simulink model "Test_Ralenti_BO_End_New"  (R2024b)
settings: Solver=ode45  StartTime=0.0  StopTime=80  FixedStep=10e-3  MaxStep=0.01  RelTol=1e-5  AbsTol=1e-6
undefined symbols (not defined in the file): AaNeTest, AirMotTest, AirPapTest, AirPressureTest, AirTimeTest, Copti, EngineSpeedTest, EngineSpeedTimeTest, NeTest, NeTimeTest, PcolNeTest, SectionBpNeTest, table_rdt_AA, TorqueLosesTest, TorqueLosesTimeTest, vect_delta_AA
settings Model: Creator=a030141  LastModifiedBy=ramse
settings SolverCC: AutoScaleAbsTol=off  AlgebraicLoopSolver=TrustRegion
settings DataIOCC: SaveFormat=Array  SignalLoggingSaveFormat=ModelDataLogs  ReturnWorkspaceOutputs=off  SignalLoggingName=sigsOut
settings OptimizationCC: BlockReduction=off  BooleanDataType=off  InitFltsAndDblsToZero=on  LifeSpan=inf
settings DebuggingCC: SaveWithParameterizedLinksMsg=none  UnderspecifiedInitializationDetection=Classic  MergeDetectMultiDrivingBlocksExec=none  SignalResolutionControl=TryResolveAllWithWarning  MultiTaskDSMMsg=warning  MultiTaskCondExecSysMsg=none  FcnCallInpInsideContextMsg=warning  UnconnectedInputMsg=warning  UnconnectedOutputMsg=warning  UnconnectedLineMsg=warning  SFUnexpectedBacktrackingDiag=warning  SFNoUnconditionalDefaultTransitionDiag=warning  SFExecutionAtInitializationDiag=none  ArithmeticOperatorsInVariantConditions=warning
settings HardwareCC: ProdBitPerPointer=32  ProdBitPerSizeT=32  ProdBitPerPtrDiffT=32  ProdLargestAtomicFloat=None  ProdIntDivRoundTo=Undefined  ProdEndianess=Unspecified  ProdWordSize=32  ProdHWDeviceType=32-bit Generic  TargetUnknown=on
settings ModelReferenceCC: PropagateSignalLabelsOutOfModel=off
settings RTWCC: TemplateMakefile=grt_vc.tmf  GPUComputeCapability=3.5
settings CodeAppCC: StateflowObjectComments=on
settings GRTTargetCC: TargetFcnLib=ansi_tfl_tmw.mat  TargetLangStandard=C89/C90 (ANSI)  CombineOutputUpdateFcns=off  GRTInterface=on
settings ConfigComp: CovMetricSettings=dw  CovSaveCumulativeToWorkspaceVar=on  CovSaveSingleToWorkspaceVar=on

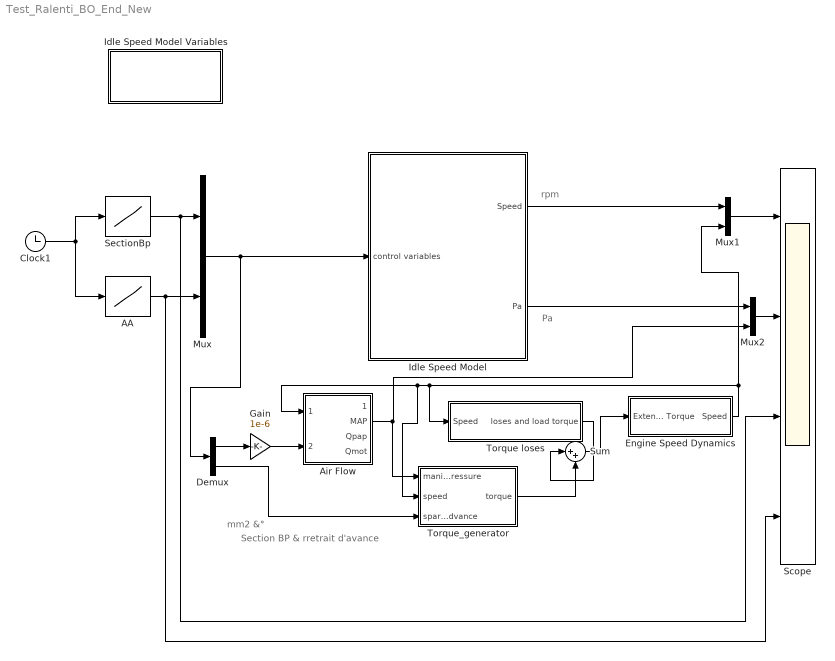
== system Test_Ralenti_BO_End_New ==
  note: Section BP & rretrait d'avance
  note: Pa
  note: rpm
  note: mm2 &°
  " Torque loses" : Subsystem
  AA : Lookup  InputValues=NeTimeTest  Table=AaNeTest
  Air Flow : Subsystem
  Clock1 : Clock
  Demux : Demux  Outputs=2
  Engine Speed Dynamics : Subsystem
  Gain : Gain  Gain=1e-6
  Idle Speed Model : Subsystem
      mask Display: disp('ENGINE MODEL\nLF -> event stroke')
  Idle Speed Model Variables : Subsystem
      mask Display: disp('Load\nDisturbances')
  Mux : Mux  Inputs=2
  Mux1 : Mux  Inputs=2
  Mux2 : Mux  Inputs=2
  Scope : Scope  NumInputPorts=4
  SectionBp : Lookup  InputValues=NeTimeTest  Table=SectionBpNeTest
  Sum : Sum  Inputs=|++
  Torque_generator : Subsystem
  wires:
  Mux/1 -> Demux/1, Idle Speed Model/1(control variables)
  SectionBp/1 -> Mux/1, Scope/3
  AA/1 -> Mux/2, Scope/4
  Clock1/1 -> SectionBp/1, AA/1
  Idle Speed Model/1(Speed) -> Mux1/1
  Mux1/1 -> Scope/1
  Idle Speed Model/2(Pa) -> Mux2/1
  Mux2/1 -> Scope/2
  Air Flow/2(MAP) -> Torque_generator/1(manifold pressure), Mux2/2
  Demux/1 -> Gain/1
  Gain/1 -> Air Flow/2(Bypass)
  Demux/2 -> Torque_generator/3(spark advance)
  Torque_generator/1(torque) -> Sum/2
  " Torque loses"/1(loses and load torque) -> Sum/1
  Sum/1 -> Engine Speed Dynamics/1(Extended Torque)
  Engine Speed Dynamics/1(Speed) -> " Torque loses"/1(Speed), Torque_generator/2(speed), Air Flow/1(Speed), Mux1/2

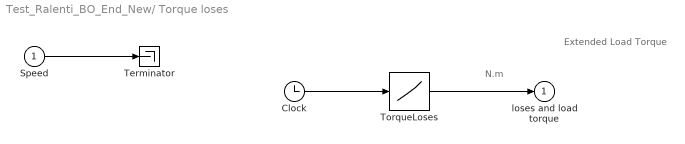
== system Test_Ralenti_BO_End_New/ Torque loses ==
  note: N.m
  note: Extended Load Torque
  Speed : Inport
  Clock : Clock
  Terminator : Terminator
  TorqueLoses : Lookup  InputValues=TorqueLosesTimeTest  Table=TorqueLosesTest
  loses and load torque : Outport
  wires:
  Clock/1 -> TorqueLoses/1
  TorqueLoses/1 -> loses and load torque/1
  Speed/1 -> Terminator/1

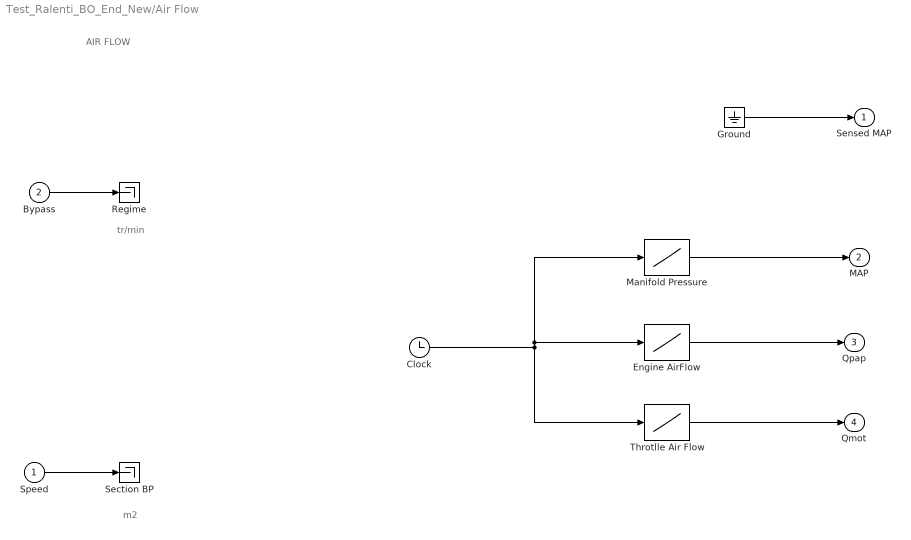
== system Test_Ralenti_BO_End_New/Air Flow ==
  note: AIR FLOW
  note: m2
  note: tr/min
  Speed : Inport
  Bypass : Inport  Port=2
  Clock : Clock
  Engine AirFlow : Lookup  InputValues=AirTimeTest  Table=AirMotTest
  Ground : Ground
  Manifold Pressure : Lookup  InputValues=AirTimeTest  Table=AirPressureTest
  Regime : Terminator
  Section BP : Terminator
  Throtlle Air Flow : Lookup  InputValues=AirTimeTest  Table=AirPapTest
  Sensed MAP : Outport
  MAP : Outport  Port=2
  Qpap : Outport  Port=3
  Qmot : Outport  Port=4
  wires:
  Bypass/1 -> Regime/1
  Speed/1 -> Section BP/1
  Ground/1 -> Sensed MAP/1
  Clock/1 -> Manifold Pressure/1, Engine AirFlow/1, Throtlle Air Flow/1
  Manifold Pressure/1 -> MAP/1
  Throtlle Air Flow/1 -> Qmot/1
  Engine AirFlow/1 -> Qpap/1

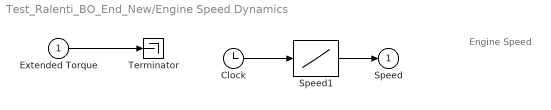
== system Test_Ralenti_BO_End_New/Engine Speed Dynamics ==
  note: Engine Speed
  Extended Torque : Inport
  Clock : Clock
  Speed1 : Lookup  InputValues=EngineSpeedTimeTest  Table=EngineSpeedTest
  Terminator : Terminator
  Speed : Outport
  wires:
  Speed1/1 -> Speed/1
  Clock/1 -> Speed1/1
  Extended Torque/1 -> Terminator/1

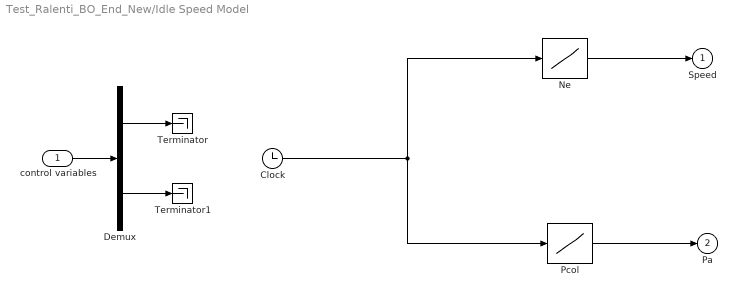
== system Test_Ralenti_BO_End_New/Idle Speed Model ==
  control variables : Inport
  Clock : Clock
  Demux : Demux  Outputs=2
      settings: DisplayOption=none
  Ne : Lookup  InputValues=NeTimeTest  Table=NeTest
  Pcol : Lookup  InputValues=NeTimeTest  Table=PcolNeTest
  Terminator : Terminator
  Terminator1 : Terminator
  Speed : Outport
  Pa : Outport  Port=2
  wires:
  Demux/1 -> Terminator/1
  control variables/1 -> Demux/1
  Ne/1 -> Speed/1
  Pcol/1 -> Pa/1
  Clock/1 -> Ne/1, Pcol/1
  Demux/2 -> Terminator1/1

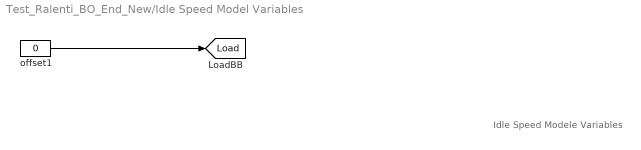
== system Test_Ralenti_BO_End_New/Idle Speed Model Variables ==
  note: Idle Speed Modele Variables
  offset1 : Constant  Value=0
  tag scope: Load=global
  wires:
  offset1/1 -> [Load]

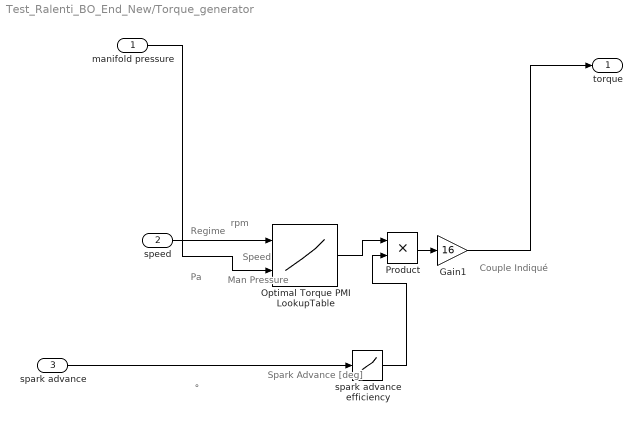
== system Test_Ralenti_BO_End_New/Torque_generator ==
  note: Regime
  note: Couple Indiqué
  note: rpm
  note: Pa
  note: °
  note: Man Pressure
  note: Speed
  note: Spark Advance
      | [deg]
  manifold pressure : Inport
  speed : Inport  Port=2
  spark advance : Inport  Port=3
  Gain1 : Gain  Gain=16
  Optimal Torque PMI LookupTable : Lookup2D  RowIndex=Ne_remp  ColumnIndex=Pcol_remp  Table=Copti
  Product : Product
  spark advance efficiency : Lookup  InputValues=vect_delta_AA  Table=table_rdt_AA
  torque : Outport
  wires:
  Product/1 -> Gain1/1
  spark advance efficiency/1 -> Product/2
  speed/1 -> Optimal Torque PMI LookupTable/1
  manifold pressure/1 -> Optimal Torque PMI LookupTable/2
  Gain1/1 -> torque/1
  Optimal Torque PMI LookupTable/1 -> Product/1
  spark advance/1 -> spark advance efficiency/1
